simulink model "mpu6050_gyro_modelling"  (R2022b)
settings: Solver=VariableStepAuto  StartTime=0.0  StopTime=10.0  RelTol=1e-3
values from neighbouring files (symbols this model uses):
  w = 0.9    [PI_tuning_using_PSO_2nd_order.m]
  wn = 5    [transient_response_analysis.m]
  z = [0]    [bode.m]    (also in nyquist.m; transient_response_analysis.m = lsim(sys, r, t))
  zeta = [0 0.2 0.4 0.6 0.8 1]    [transient_response_analysis.m]
undefined symbols (not defined in the file or in its folder): Bias
libraries: simulink x1
settings Model: Creator=SIDDHARTH  LastModifiedBy=SIDDHARTH

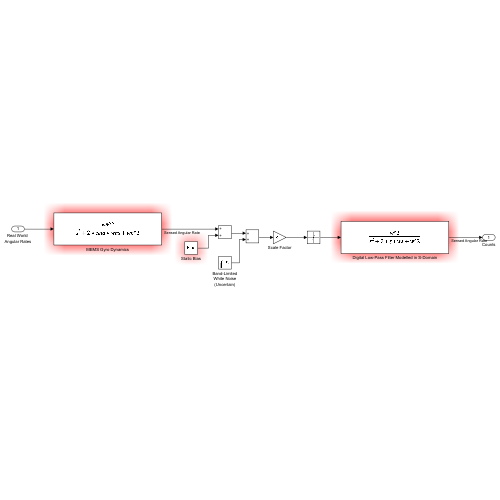
[thumbnail: Simulink's stored preview of the top-level diagram]
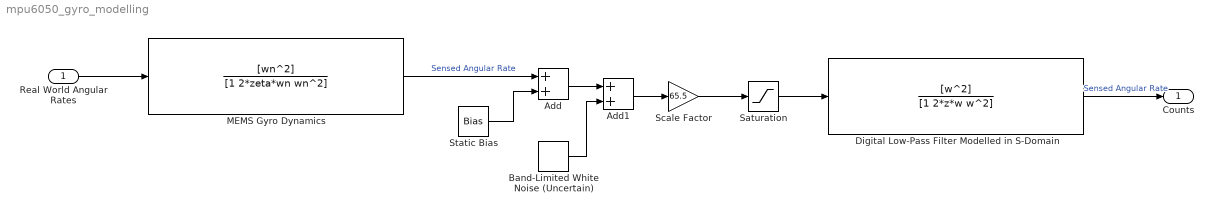
== system mpu6050_gyro_modelling ==
  Real World Angular Rates : Inport
  Add : Sum
  Add1 : Sum
  Band-Limited White Noise (Uncertain) : simulink/Sources/Band-Limited White Noise  Cov=[0.005^2]  Ts=1/1000  seed=[23341]
  Digital Low-Pass Filter Modelled in S-Domain : TransferFcn  Numerator=[w^2]  Denominator=[1 2*z*w w^2]
  MEMS Gyro Dynamics : TransferFcn  Numerator=[wn^2]  Denominator=[1 2*zeta*wn wn^2]
  Saturation : Saturate  UpperLimit=2^15  LowerLimit=-2^15
  "Scale Factor " : Gain  Gain=65.5
  Static Bias : Constant  Value=Bias
  Counts : Outport
  wires:
  Real World Angular Rates/1 -> MEMS Gyro Dynamics/1
  "Scale Factor "/1 -> Saturation/1
  MEMS Gyro Dynamics/1 -> Add/1  "Sensed Angular Rate"
  Static Bias/1 -> Add/2
  Add/1 -> Add1/1
  Band-Limited White Noise (Uncertain)/1 -> Add1/2
  Add1/1 -> "Scale Factor "/1
  Saturation/1 -> Digital Low-Pass Filter Modelled in S-Domain/1
  Digital Low-Pass Filter Modelled in S-Domain/1 -> Counts/1  "Sensed Angular Rate"
